simulink model "V1_Ball_and_Bean_Controller"  (R2014a)
settings: Solver=ode4  SolverMode=SingleTasking  StartTime=0.0  StopTime=Inf  FixedStep=0.0001  RelTol=1e-3
PostLoadFcn:
  | , if any(exist('dsrtsu_mdlpostloadfcn', 'file') == [2, 3, 6]), try dsrtsu_mdlpostloadfcn('Execute', bdroot); catch fprintf('Error in PostLoadFcn (dsrtsu_mdlpostloadfcn) for model "%s":\n %s\n', bdroot, lasterr); end, end,
libraries: rtilib1104 x2
settings Model: DSRTSU_INTERNAL_RTI_VER=450  DSRTSU_INTERNAL_RTI_TYPE=rti1104  RTICANMMDATA=struct('GeneralSetupData',struct('modelroot','I:\ChristianeB\FürDorsa\Sandbox_RTI_Demos\Model\DS1104\Model','generalsettings',struct('filesettings',struct('destfolder',struct('Name','RTICANMM_FILES','Check',1),'buildfolder',struct('Name','.','Check',1),'AbsDestfolder',struct('Name','I:\ChristianeB\FürDorsa\Sandbox_RTI_Demos\Model\DS1104\Model\RTICANMM_FILES'),'AbsBuildfolder',struct('Name','I:\ChristianeB\FürDorsa\Sandbox_RTI_Demos\Model\DS1104\Model'))),'options',struct('addpaths',1,'rmpaths',1,'addtrcexclusion',logical(1),'cannavigator',struct('checkmonitoring',0),'show_usrtrc',0,'use_usrtrc',0),'advanced',struct('options',[1 1 1 1 1 1 1 1 1 1 1 1 1 1 1 1 1 1 1 1 1 1 1 1 1 1 1 1 1 1 1 1 1 1 1 1 1 1 1 1 1 1 1 1 1 1 1 1 1 1 1 1 1 1 1 1 1 1 1 1 1 1 1 1 1 1 1 1 1 1 1 1 1 1 1 1 1 1 1 1 1 1 1 1 1 1 1 1 1 1 1 1 1 1 1 1 1 1 1 1]),'MPSetup',{{}},'modelname','demo1104_timerio1','block','demo1104_timerio1'))  DSRTSU_INTERNAL_RTIFLEXRAYCONFIG=50  DSRTSU_INTERNAL_RTIFPGA=40  ExtModeTrigMode=oneshot  ExtModeArmWhenConnect=off  BufferReuse=off  Creator=dSPACE GmbH  LastModifiedBy=Usuario
settings DataIOCC: SignalLoggingSaveFormat=ModelDataLogs
settings OptimizationCC: BlockReduction=off  ConditionallyExecuteInputs=off  OptimizeBlockIOStorage=off  BufferReuse=off  GlobalBufferReuse=off  ExpressionFolding=off  ExpressionDepthLimit=2147483647  LocalBlockOutputs=off  InitFltsAndDblsToZero=on
settings DebuggingCC: SaveWithParameterizedLinksMsg=none  UnderspecifiedInitializationDetection=Classic  SignalResolutionControl=TryResolveAllWithWarning  MultiTaskDSMMsg=warning  MultiTaskCondExecSysMsg=none  MultiTaskRateTransMsg=warning  TasksWithSamePriorityMsg=none  FcnCallInpInsideContextMsg=UseLocalSettings  StateNameClashWarn=warning
settings HardwareCC: ProdIntDivRoundTo=Zero  ProdEndianess=BigEndian  ProdHWDeviceType=Generic->Custom  TargetIntDivRoundTo=Zero  TargetEndianess=BigEndian  TargetHWDeviceType=Generic->Custom
settings RTWCC: SystemTargetFile=rti1104.tlc  MakeCommand=make_rti  TemplateMakefile=rti1104.tmf  Description=dSPACE DS1104 Hardware Platform  RTWVerbose=off  ProcessScript=rti1104_make_rtw_hook  IncludeERTFirstTime=on
settings STFCustomTargetCC: TargetFcnLib=ansi_tfl_tmw.mat  ParMdlRefBuildCompliant=on  ConcurrentExecutionCompliant=off  SystemTargetFile=rti1104.tlc
settings GRTTargetCC: TargetFcnLib=ansi_tfl_tmw.mat  CompOptLevelCompliant=off  ConcurrentExecutionCompliant=off  CombineOutputUpdateFcns=off  MatFileLogging=off  CPPClassGenCompliant=off  GRTInterface=on  ExtModeMexFile=noextcomm

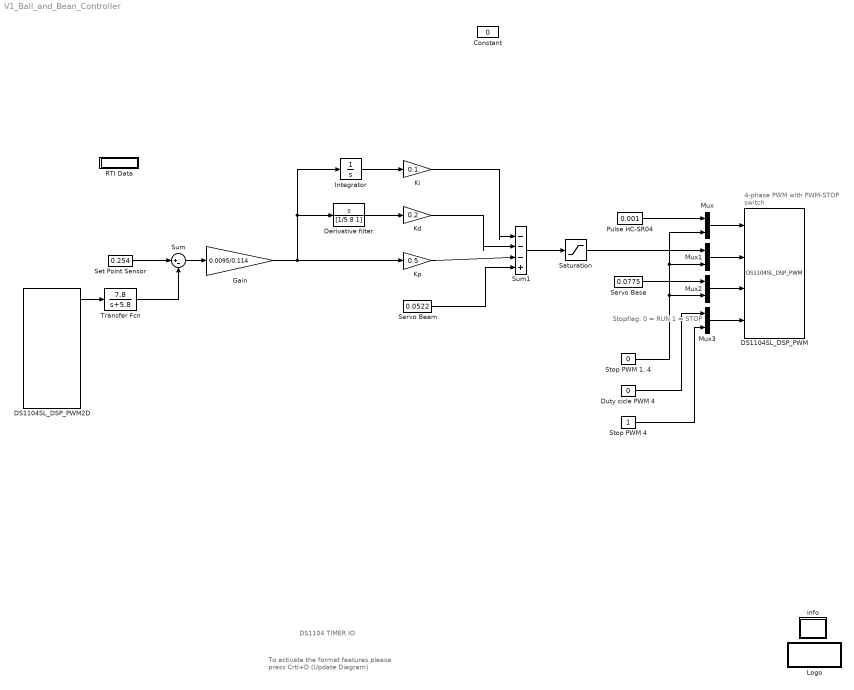
== system V1_Ball_and_Bean_Controller ==
  note: 4-phase PWM with
      | PWM-STOP switch
  note: Stopflag:
      | 0 = RUN
      | 1 = STOP
  note: To activate the format features please
      | press Crtl+D (Update Diagram)
  note: DS1104 TIMER IO
  Constant : Constant  Value=0
  DS1104SL_DSP_PWM : rtilib1104/DS1104 SLAVE DSP/DS1104SL_DSP_PWM  Parameters=[]  TDef=[]  BoardType=[]  PwmMode=[]  Frequency=[]  InitValue=[]  TermMode=[]  TermValue=[]  Polarity=[]  DialogFcn=[]  Reserved1=[]  Reserved2=[]  Reserved3=[]  Reserved4=[]  Revision=[]  UnitName=[]  UnitValues=[]  DSProperties=struct('RTI',struct('Version',uint32(2),'BlockType',struct('isSLSource',uint8(0),'isSLSink',uint8(1),'isHWSource',uint8(0),'isHWSink',uint8(1),'isSetup',uint8(0),'isInline',uint8(1),'isNonInline',uint8(0),'isInterrupt',uint8(0),'isChannelwise',uint8(0)),'IOBoardType','DS1104SLAVE','UnitType','PWM','Identifier','PWM','DialogType','ML','BlockSet','NONE','SlaveProcessor','F240'))  RTIBlockInterface=struct('InputPortsActive',[1 1 1 1],'InputPortsWidth',int32([2 2 2 2]),'InputPortsName',{{['PWM Channel 1'],['PWM Channel 2'],['PWM Channel 3'],['PWM Channel 4']}},'IWork',{{{'',uint32(4)}}},'DialogFcn','rti1104slavepwmgui','InitLevel',1,'BlockDisplay',{{'','auto'}},'IconTransparency','on','MultiSFcn',4,'BlockName',struct('Token',{{'DS1104SL_DSP_PWM'}}))  RTIBlockParameters=struct('PWMSymmetryMode',{{2,'OFF',[]}},'PWMFrequency',{{'50','OFF',[]}},'PWMPolarityMode',{{[1 1 1 1 1],'OFF',[]}},'ChannelNo',{{[1 2 3 4],'OFF',[]}},'SuspendModeInit',{{[1 1 1 1 1],'OFF',[]}},'TTLModeInit',{{[2 2 2 2 2],'OFF',[]}},'DutyCycleInitValueCh1',{{'0.5','OFF',[]}},'DutyCycleInitValueCh2',{{'0.5','OFF',[]}},'DutyCycleInitValueCh3',{{'0.5','OFF',[]}},'DutyCycleInitValueCh4',{{'0.5','OFF',[]}},'DutyCycleInitValueCh5',{{'0.5','OFF',[]}},'EnablePWMStop',{{[1 1 1 1 0],'OFF',[]}},'SuspendModeTerm',{{[1 1 1 1 1],'OFF',[]}},'TTLModeTerm',{{[2 2 2 2 2],'OFF',[]}},'DutyCycleTermValueCh1',{{'0.5','OFF',[]}},'DutyCycleTermValueCh2',{{'0.5','OFF',[]}},'DutyCycleTermValueCh3',{{'0.5','OFF',[]}},'DutyCycleTermValueCh4',{{'0.5','OFF',[]}},'DutyCycleTermValueCh5',{{'0.5','OFF',[]}},'TLCFileName',{{'rti1104pwm','OFF',[]}})  RTISFcnParameters=struct('PWMSymmetryMode','double','PWMFrequency','double','PWMPolarityMode','double','ChannelNo','double','SuspendModeInit','double','TTLModeInit','double','DutyCycleInitValueCh1','double','DutyCycleInitValueCh2','double','DutyCycleInitValueCh3','double','DutyCycleInitValueCh4','double','EnablePWMStop','double','SuspendModeTerm','double','TTLModeTerm','double','DutyCycleTermValueCh1','double','DutyCycleTermValueCh2','double','DutyCycleTermValueCh3','double','DutyCycleTermValueCh4','double','TLCFileName','char')  RTIBlockParaDefault=struct('PWMSymmetryMode',1,'PWMFrequency',100,'PWMPolarityMode',[1 1 1 1 1],'ChannelNo',[1 2 3 4],'SuspendModeInit',[1 1 1 1 1],'TTLModeInit',[2 2 2 2 2],'DutyCycleInitValueCh1',0.5,'DutyCycleInitValueCh2',0.5,'DutyCycleInitValueCh3',0.5,'DutyCycleInitValueCh4',0.5,'DutyCycleInitValueCh5',0.5,'EnablePWMStop',[1 1 1 1 0],'SuspendModeTerm',[1 1 1 1 1],'TTLModeTerm',[2 2 2 2 2],'DutyCycleTermValueCh1',0.5,'DutyCycleTermValueCh2',0.5,'DutyCycleTermValueCh3',0.5,'DutyCycleTermValueCh4',0.5,'DutyCycleTermValueCh5',0.5,'TLCFileName','rti1104pwm')
  DS1104SL_DSP_PWM2D : rtilib1104/DS1104 SLAVE DSP/DS1104SL_DSP_PWM2D  Reserved1=[]  Reserved2=[]  Reserved3=[]  Reserved4=[]  DialogFcn=gui1104sl_dsp_pwm2d  UnitName={'DS1104SL_DSP_PWM2D'}  UnitValues={ [] }  DSProperties=struct('RTI',struct('Version',uint32(1),'BlockType',struct('isSLSource',uint8(1),'isSLSink',uint8(0),'isHWSource',uint8(1),'isHWSink',uint8(0),'isSetup',uint8(0),'isInline',uint8(1),'isNonInline',uint8(0),'isInterrupt',uint8(0),'isChannelwise',uint8(0)),'IOBoardType','DS1104SLAVE','UnitType','PWM','Identifier','PWM2D','DialogType','ML','BlockSet','NONE','SlaveProcessor','F240'))
  Derivative filter : TransferFcn  Numerator=[1 0]  Denominator=[1/5.8 1]
  Duty cicle PWM 4 : Constant  Value=0  OutDataTypeStr=double
  Gain : Gain  Gain=0.0095/0.114
  Integrator : Integrator
  Kd : Gain  Gain=0.2  SaturateOnIntegerOverflow=on  OutDataTypeStr=Inherit: Same as input  ParamDataTypeStr=Inherit: Same as input
  Ki : Gain  Gain=0.1  SaturateOnIntegerOverflow=on  OutDataTypeStr=Inherit: Same as input  ParamDataTypeStr=Inherit: Same as input
  Kp : Gain  Gain=0.5  SaturateOnIntegerOverflow=on  OutDataTypeStr=Inherit: Same as input  ParamDataTypeStr=Inherit: Same as input
  Logo : Subsystem  mask(dSPACE){EmptyParameter=[]}
      mask prompts: EmptyParameter "Mask Parameter 1:"
      settings: OpenFcn=;
      mask Display: image(imread('rti_mdl_dslogo.tif'));
  Mux{,1..3} (4 alike) : Mux  Inputs=2
  Pulse HC-SR04 : Constant  Value=0.001  OutMin=[0]  OutMax=[0.1]  OutDataTypeStr=double
  RTI Data : Subsystem  Tag=struct('RTIDataServer',struct('RTIDataServerVs','2','RTIModelDescription','struct(''main'',''V1_Ball_and_Bean_Controller'',''sub'','''',''isMp'',0)'))  LoadFcn="if exist('rtidc'), try,  rtidc('DataHostBlockClbLoad', gcbh); catch, disp(['Warning: ''LoadFcn'' for RTI Data block failed: ' lasterr]); end, end,"  mask(RTI_DATA_HOST){}
      mask help:
      | RTI Data Block.
      | This block is used by RTI to store internal model-dependent data.
      | Please keep this block on the root level of the model. Deleting this block will result in data loss.
      |
      | NEVER DELETE OR COPY THIS BLOCK!
      settings: CopyFcn="if exist('rtidc'), try,  rtidc('DataHostBlockClbCopy', gcbh); catch, disp(['Warning: ''CopyFcn'' for RTI Data block failed: ' lasterr]); end, end,"  DeleteFcn="if exist('rtidc'), try,  rtidc('DataHostBlockClbDelete', gcbh); catch, disp(['Warning: ''DeleteFcn'' for RTI Data block failed: ' lasterr]); end, end,"  ModelCloseFcn="if exist('rtidc'), try,  rtidc('DataHostBlockClbModelClose', gcbh); catch, disp(['Warning: ''ModelCloseFcn'' for RTI Data block failed: ' lasterr]); end, end,"  PreSaveFcn="if exist('rtidc'), try,  rtidc('DataHostBlockClbPreSave', gcbh); catch, disp(['Warning: ''PreSaveFcn'' for RTI Data block failed: ' lasterr]); end, end,"  PostSaveFcn="if exist('rtidc'), try,  rtidc('DataHostBlockClbPostSave', gcbh); catch, disp(['Warning: ''PostSaveFcn'' for RTI Data block failed: ' lasterr]); end, end,"  NameChangeFcn="if exist('rtidc'), try,  rtidc('DataHostBlockClbNameChange', gcbh); catch, disp(['Warning: ''NameChangeFcn'' for RTI Data block failed: ' lasterr]); end, end,"
      mask Help:
      | RTI Data Block.
      | This block is used by RTI to store internal model-dependent data.
      | Please keep this block on the root level of the model. Deleting this block will result in data loss.
      | 
      | NEVER DELETE OR COPY THIS BLOCK!
      mask Display:
      | text(0.5, 0.5, 'RTI Data', 'HorizontalAlignment', 'center');
      | plot([1 0]);
  Saturation : Saturate  UpperLimit=0.0617  LowerLimit=0.0427  OutMin=[0.0427]  OutMax=[0.0617]  OutDataTypeStr=double
  Servo Base : Constant  Value=0.0775  OutMin=[0.0750]  OutMax=[0.08]
  Servo Beam : Constant  Value=0.0522  OutMin=[0.0390]  OutMax=[0.0580]
  Set Point Sensor : Constant  Value=0.254  OutMin=[0.03]  OutMax=[0.55]  OutDataTypeStr=double
  Stop PWM 1..4 : Constant  Value=0
  Stop PWM 4 : Constant  OutDataTypeStr=double
  Sum : Sum  Inputs=|+-
  Sum1 : Sum  Inputs=|---+
  Transfer Fcn : TransferFcn  Numerator=[7.8]  Denominator=[1 5.8]
  info : Subsystem
      mask Display: disp('?')
  wires:
  Mux/1 -> DS1104SL_DSP_PWM/1
  Stop PWM 1..4/1 -> Mux/2, Mux1/2, Mux2/2
  Mux1/1 -> DS1104SL_DSP_PWM/2
  Mux2/1 -> DS1104SL_DSP_PWM/3
  Mux3/1 -> DS1104SL_DSP_PWM/4
  Saturation/1 -> Mux1/1
  Servo Base/1 -> Mux2/1
  Set Point Sensor/1 -> Sum/1
  Sum/1 -> Gain/1
  Sum1/1 -> Saturation/1
  Transfer Fcn/1 -> Sum/2
  Gain/1 -> Kp/1, Integrator/1, Derivative filter/1
  Derivative filter/1 -> Kd/1
  Integrator/1 -> Ki/1
  Servo Beam/1 -> Sum1/4
  Pulse HC-SR04/1 -> Mux/1
  Stop PWM 4/1 -> Mux3/2
  Duty cicle PWM 4/1 -> Mux3/1
  DS1104SL_DSP_PWM2D/1 -> Transfer Fcn/1
  Ki/1 -> Sum1/1
  Kd/1 -> Sum1/2
  Kp/1 -> Sum1/3

== system V1_Ball_and_Bean_Controller/Logo ==
  note: $Revision: 2.6 $
  note: $Date: 2013/07/08 18:15:06MESZ $
  note: $RCSfile: demo1104_timerio1.mdl $

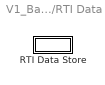
== system V1_Ball_and_Bean_Controller/RTI Data ==
  RTI Data Store : Subsystem  Tag="struct('private',struct('version',struct('dsVer',uint32(2),'dsVerCreation',uint32(2),'RTI',struct('ver','7.3','type','RTI1104')),'access',struct('type','Model','isPerm',1,'created',['08-Sep-2022 09:36:06'],'modified',['13-Sep-2022 12:03:05'],'location','')),'public',struct('main',struct('data',[]),'sub',struct('name',{{'V1_Ball_and_Bean_Controller'}},'data',{{struct('TH',struct('thTaskInfo',struct('taskType',{'TIMER','HWINT','TMRINT','SWINT','GLINT'},'tasksNumOf',{1,0,0,0,0},'srcIds',{{'TIMERA'},{},{},{},{}},'taskNames',{{['Timer Task 1']},{},{},{},{}})),'th_tc',struct('dataType','TASK','taskGroupId','','taskGroupList',{{}},'taskSchedulingPolicy','FCFS','taskType','TIMER','blkh',-1,'srcId','TIMERA','srcSgnName',['Timer A interrupt'],'srcCpuName','','taskName',['Timer Task 1  [0.0001] s'],'taskNameDisplayExt','','smplTime',0.0001,'smplTimeOffs',0,'hasFixedPriority',0,'priority',1,'hasFixedOvc',0,'ovcType',1,'ovcMax',1),'tc_th',struct('dataType','TASK','taskGroupId','','taskGroupList',{{}},'taskSchedulingPolicy','FCFS','taskType','TIMER','blkh',-1,'srcId','TIMERA','srcSgnName',['Timer A interrupt'],'srcCpuName','','taskName',['Timer Task 1  [0.0001] s'],'taskNameDisplayExt','','smplTime',0.0001,'smplTimeOffs',0,'hasFixedPriority',0,'priority',1,'hasFixedOvc',0,'ovcType',1,'ovcMax',1))}})))"  mask(RTI_DATA_STORE){}
      mask help:
      | RTI Data Store Block. This block is used by RTI to store internal model dependent data. Deleting this block will result in data loss.
      |
      | NEVER DELETE, COPY, OR MODIFY THIS BLOCK!
      mask Help:
      | RTI Data Store Block. This block is used by RTI to store internal model dependent data. Deleting this block will result in data loss.
      | 
      | NEVER DELETE, COPY, OR MODIFY THIS BLOCK!
      mask Display: text(0.5, 0.5, ' ', 'HorizontalAlignment', 'center');

== system V1_Ball_and_Bean_Controller/info ==
  note: Objective:
      |
      | To demonstrate the behavior of the timer I/O units which are supported by RTI.
      |
      |
      | Basic information on the DS1104 Board:
      |
      | The Real-Time Interface (RTI) board library for the DS1104 R&D Controller Board,
      |  rtilib1104, provides the RTI blocks that implement the I/O capabilities of the DS1104
      |  in Simulink models.
      | These RTI blocks are designed to specify the hardware setup for real-time applications.
      | rtilib1104 also provides additional RTI blocks, demo models, and useful information.
      |
      |
      |
      | In this demo:
      |
      | DS1104SL_DSP_PWM -> To write to a single bit of the 20-bit digital output.
      | DS1104SL_DSP_PWM2D -> To measure the duty cycles and the frequencies
      | from up to 4 independent channels used for PWM-type signals..
      |
      |
      |
      | Note:
      |
      | After building and downloading the model (<Crtl-B>) to the DS1104,
      | you can watch the output signals of the PWMsignal generator PWM on an oscilloscope.
      | Connect outputs ST2PWM, SPWM7, SPWM8 or SPWM9 to the oscilloscope.
      | The four generated PWM signals are center aligned.
      | To measure their frequencies and duty cycles with the PWM2D block,
      | connect the above-mentioned outputs with inputs SCAP1 to SCAP4.
      | You can watch the results in ControlDesk.
      |
      | For information on an RTI block, double-click the board button.
      | Click Help to navigate to the Block description in dSPACE HelpDesk.

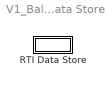
== system V1_Ball_and_Bean_Controller/RTI Data/RTI Data Store ==
  RTI Data Store : Subsystem  mask(RTI_DATA_STORE){}
      mask help:
      | RTI Data Store Block. This block is used by RTI to store internal model dependent data. Deleting this block will result in data loss.
      |
      | NEVER DELETE, COPY, OR MODIFY THIS BLOCK!
      mask Help:
      | RTI Data Store Block. This block is used by RTI to store internal model dependent data. Deleting this block will result in data loss.
      | 
      | NEVER DELETE, COPY, OR MODIFY THIS BLOCK!
      mask Display: text(0.5, 0.5, ' ', 'HorizontalAlignment', 'center');

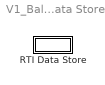
== system V1_Ball_and_Bean_Controller/RTI Data/RTI Data Store/RTI Data Store ==
  RTI Data Store : Subsystem  mask(RTI_DATA_STORE){}
      mask help:
      | RTI Data Store Block. This block is used by RTI to store internal model dependent data. Deleting this block will result in data loss.
      |
      | NEVER DELETE, COPY, OR MODIFY THIS BLOCK!
      mask Help:
      | RTI Data Store Block. This block is used by RTI to store internal model dependent data. Deleting this block will result in data loss.
      | 
      | NEVER DELETE, COPY, OR MODIFY THIS BLOCK!
      mask Display: text(0.5, 0.5, ' ', 'HorizontalAlignment', 'center');

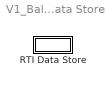
== system V1_Ball_and_Bean_Controller/RTI Data/RTI Data Store/RTI Data Store/RTI Data Store ==
  RTI Data Store : Subsystem  mask(RTI_DATA_STORE){}
      mask help:
      | RTI Data Store Block. This block is used by RTI to store internal model dependent data. Deleting this block will result in data loss.
      |
      | NEVER DELETE, COPY, OR MODIFY THIS BLOCK!
      mask Help:
      | RTI Data Store Block. This block is used by RTI to store internal model dependent data. Deleting this block will result in data loss.
      | 
      | NEVER DELETE, COPY, OR MODIFY THIS BLOCK!
      mask Display: text(0.5, 0.5, ' ', 'HorizontalAlignment', 'center');

== system V1_Ball_and_Bean_Controller/RTI Data/RTI Data Store/RTI Data Store/RTI Data Store/RTI Data Store ==
